simulink model "PiezoMPC2_17"  (R2022a)
settings: Solver=ode5  StartTime=0.0  StopTime=40  FixedStep=0.0001  RelTol=1e-3
values from neighbouring files (symbols this model uses):
  A = -1/tau    (= -1000)    [piezo_main.m]
  Abw = betas(7)    [StateFunction.m]    (also in piezo_main.m = 0.9)
  alpha = 80    [piezo_main.m]
  Aobs = [0, -B ... (first row only)    [piezo_main.m]
  B = 1/tau    (= 1000)    [piezo_main.m]
  beta1 = betas(1)    [StateFunction.m]    (also in piezo_main.m = 0.0032)
  beta2 = betas(2)    [StateFunction.m]    (also in piezo_main.m = 0.0035)
  beta3 = betas(3)    [StateFunction.m]    (also in piezo_main.m = -0.001)
  beta4 = betas(4)    [StateFunction.m]    (also in piezo_main.m = -0.0003)
  beta5 = betas(5)    [StateFunction.m]    (also in piezo_main.m = -0.0002)
  beta6 = betas(6)    [StateFunction.m]    (also in piezo_main.m = 0.0004)
  betas = [beta1;beta2;beta3;beta4;beta5;beta6;Abw;A;B;dp]    [piezo_main.m]
  C = [1, 0]    [piezo_main.m]
  dp = 1.6    [piezo_main.m]
  K = [10.0, 0.0 ... (first row only)    [piezo_main.m]
  kappa = 500    [piezo_main.m]
  S_inv = [  2*theta ,        -(1/B)*theta^2 ... (first row only)    [piezo_main.m]
undefined symbols (not defined in the file or in its folder): freq
libraries: mpclib x1
settings Model: Creator=CIO  LastModifiedBy=CIO
settings SolverCC: AlgebraicLoopSolver=TrustRegion
settings OptimizationCC: ZeroExternalMemoryAtStartup=off  ZeroInternalMemoryAtStartup=off  InitFltsAndDblsToZero=on
settings DebuggingCC: UnconnectedInputMsg=warning  UnconnectedOutputMsg=warning  UnconnectedLineMsg=warning  SFMachineParentedDataDiag=warning  ArithmeticOperatorsInVariantConditions=warning
settings HardwareCC: ProdLongLongMode=on  TargetLongLongMode=on
settings SFSimCC: CustomCodeUndefinedFunction=UseInterfaceOnly  SimTargetLang=C++
settings RTWCC: TargetLang=C++  DLArmComputeVersion=19.05
settings GRTTargetCC: TargetLangStandard=C++03 (ISO)  CodeInterfacePackaging=C++ class

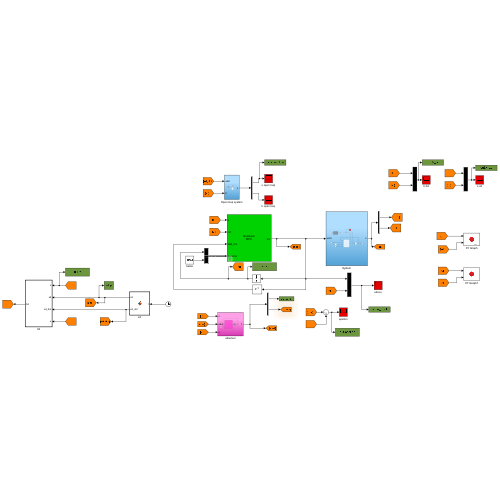
[thumbnail: Simulink's stored preview of the top-level diagram]
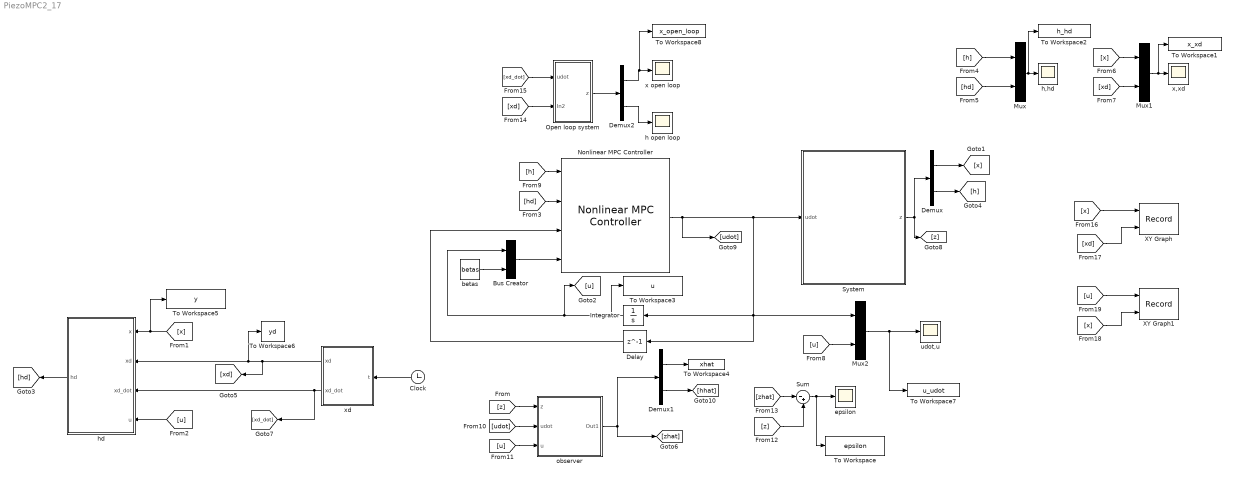
== system PiezoMPC2_17 ==
  Bus Creator : BusCreator  Inputs=2  OutDataTypeStr=Bus: myBusObject  NonVirtualBus=on
      settings: InheritFromInputs=off
  Clock : Clock
  Delay : Delay  DelayLength=1  InitialCondition=0
  Demux : Demux  Outputs=2
  Demux1 : Demux  Outputs=2
  Demux2 : Demux  Outputs=2
  Integrator : Integrator
  Mux : Mux  Inputs=2
  Mux1 : Mux  Inputs=2
  Mux2 : Mux  Inputs=2
  Nonlinear MPC Controller : mpclib/Nonlinear MPC Controller  SCDEnableBlockLinearizationSpecification=on  nlmpcobj=nlobj  UseObjectTs=on  UseMEX=off  md_enabled=off  mvtarget_enabled=off  param_enabled=on  cost_enabled=off  mvseq_enabled=off  stateseq_enabled=off  ovseq_enabled=off  slack_enabled=off  status_enabled=off  ov_min=off  ov_max=off  mv_min=off  mv_max=off  mvrate_min=off  mvrate_max=off  state_min=off  state_max=off  ov_weight=off  mv_weight=off  mvrate_weight=off  ecr_weight=off  nlp_initialize=off
  "Open loop system " : Subsystem
  Sum : Sum  Inputs=|-+
  System : Subsystem
  To Workspace : ToWorkspace  VariableName=epsilon  SampleTime=-1
  To Workspace1 : ToWorkspace  VariableName=x_xd  SampleTime=-1
  To Workspace2 : ToWorkspace  VariableName=h_hd  SampleTime=-1
  To Workspace3 : ToWorkspace  VariableName=u  SampleTime=-1
  To Workspace4 : ToWorkspace  VariableName=xhat  SampleTime=-1
  To Workspace5 : ToWorkspace  VariableName=y  SampleTime=-1
  To Workspace6 : ToWorkspace  VariableName=yd  SampleTime=-1
  To Workspace7 : ToWorkspace  VariableName=u_udot  SampleTime=-1
  To Workspace8 : ToWorkspace  VariableName=x_open_loop  SampleTime=-1
  XY Graph : Record  FileSettingsInternal="{\"entries\":[{\"content\":{\"excelSettings\":{\"content\":{},\"type\":\"Streamout.ExcelSettings\"}},\"type\":\"Streamout.FileSettingStorage\",\"uuid\":\"43ed1803-2e51-4bcb-b320-9c9d12944944\"}],\"packageUris\":[\"http://schema.mathworks.com/mf0/streamout_blocks/R2020a\"],\"version\":\"1.0\"}"  Layout=[1 1]  SignalsInternal="{\"entries\":[{\"content\":{\"signals\":[{\"content\":{\"blockPath\":[\"PiezoMPC2_17/XY Graph\"],\"channel\":[],\"dimensions\":[1],\"domain\":\"PiezoMPC2_17/XY Graph\",\"lineColor\":\"#a2142f\",\"plots\":[1],\"port\":1,\"sid\":[\"\"],\"signalID\":7776,\"signalName\":\"From16\"},\"type\":\"RecordBlkView.Signal\",\"uuid\":\"85c6ca8d-4860-42c1-af1f-82db8d25a64f\"},{\"content\":{\"blockPath\":[\"PiezoMPC2_17/XY Graph\"],\"channel\":[],\"dimensions\":[1],\"domain\":\"PiezoMPC2_17/XY Graph\",\"lineColor\":\"#139fff\",\"plots\":[1],\"port\":2,\"sid\":[\"\"],\"signalID\":7780,\"signalName\":\"From17\"},\"type\":\"RecordBlkView.Signal\",\"uuid\":\"68d22f8c-7fdf-4212-94fa-99e6d068a517\"}]},\"type\":\"RecordBlkView.InputSignals\",\"uuid\":\"7df4be47-02ba-4bd2-b1ad-eb6086c27650\"}],\"packageUris\":[\"http://schema.mathworks.com/mf0/streamout_blocks/R2020a\"],\"version\":\"1.0\"}"  VisualizationBindings="{\"xyplotplugin\":{\"info\":[{\"series\":[{\"bindingParametersList\":[{\"parameter\":\"X-Axis\",\"signalID\":7776,\"signalName\":\"From16\"},{\"parameter\":\"Y-Axis\",\"signalID\":7780,\"signalName\":\"From17\"}],\"seriesID\":32554}],\"subplotID\":1}]}}"  CompatibilityTag=XY
  XY Graph1 : Record  FileSettingsInternal="{\"entries\":[{\"content\":{\"excelSettings\":{\"content\":{},\"type\":\"Streamout.ExcelSettings\"}},\"type\":\"Streamout.FileSettingStorage\",\"uuid\":\"9b7f80d8-412e-4e2a-8833-cd9c8851424c\"}],\"packageUris\":[\"http://schema.mathworks.com/mf0/streamout_blocks/R2020a\"],\"version\":\"1.0\"}"  Layout=[1 1]  SignalsInternal="{\"entries\":[{\"content\":{\"signals\":[{\"content\":{\"blockPath\":[\"PiezoMPC2_17/XY Graph1\"],\"channel\":[],\"dimensions\":[1,1],\"domain\":\"PiezoMPC2_17/XY Graph1\",\"lineColor\":\"#a2142f\",\"plots\":[1],\"port\":1,\"sid\":[\"\"],\"signalID\":7784,\"signalName\":\"From19\"},\"type\":\"RecordBlkView.Signal\",\"uuid\":\"d37f6522-71ed-4229-9050-82b4d9bbd21d\"},{\"content\":{\"blockPath\":[\"PiezoMPC2_17/XY Graph1\"],\"channel\":[],\"dimensions\":[1],\"domain\":\"PiezoMPC2_17/XY Graph1\",\"lineColor\":\"#139fff\",\"plots\":[1],\"port\":2,\"sid\":[\"\"],\"signalID\":7788,\"signalName\":\"From18\"},\"type\":\"RecordBlkView.Signal\",\"uuid\":\"deba607d-0966-4bfa-aa24-ff5771058220\"}]},\"type\":\"RecordBlkView.InputSignals\",\"uuid\":\"5f0caead-39a7-4f6e-b661-079760aac763\"}],\"packageUris\":[\"http://schema.mathworks.com/mf0/streamout_blocks/R2020a\"],\"version\":\"1.0\"}"  VisualizationBindings="{\"xyplotplugin\":{\"info\":[{\"series\":[{\"bindingParametersList\":[{\"parameter\":\"X-Axis\",\"signalID\":7784,\"signalName\":\"From19\"},{\"parameter\":\"Y-Axis\",\"signalID\":7788,\"signalName\":\"From18\"}],\"seriesID\":21478}],\"subplotID\":1}]}}"  CompatibilityTag=XY
  betas : Constant  Value=betas  VectorParams1D=off
  epsilon : Scope
  h open loop : Scope
  h,hd : Scope
  hd : MATLAB Function  TreatAsAtomicUnit=on
  observer : Subsystem
  udot,u : Scope
  x open loop : Scope
  x,xd : Scope
  xd : MATLAB Function  TreatAsAtomicUnit=on
  wires:
  Bus Creator/1 -> Nonlinear MPC Controller/4
  betas/1 -> Bus Creator/2
  Nonlinear MPC Controller/1 -> Integrator/1, Mux2/1, Delay/1, System/1(udot), [udot]
  Delay/1 -> Nonlinear MPC Controller/3
  Integrator/1 -> To Workspace3/1, [u], Bus Creator/1
  System/1(z) -> Demux/1, [z]
  xd/2(xd_dot) -> [xd_dot], hd/3(xd_dot)
  xd/1(xd) -> [xd], To Workspace6/1, hd/2(xd)
  Clock/1 -> xd/1(t)
  [x] -> To Workspace5/1, hd/1(x)
  [u] -> hd/4(u)
  hd/1(hd) -> [hd]
  [h] -> Mux/1
  [hd] -> Mux/2
  Mux/1 -> To Workspace2/1, h,hd/1
  Mux1/1 -> To Workspace1/1, x,xd/1
  [x] -> Mux1/1
  [xd] -> Mux1/2
  Mux2/1 -> To Workspace7/1, udot,u/1
  [u] -> Mux2/2
  Demux/2 -> [h]
  Demux/1 -> [x]
  [h] -> Nonlinear MPC Controller/1
  [hd] -> Nonlinear MPC Controller/2
  [udot] -> observer/2(udot)
  [z] -> observer/1(z)
  observer/1(Out1) -> Demux1/1, [zhat]
  [u] -> observer/3(u)
  Demux1/1 -> To Workspace4/1
  Demux1/2 -> [hhat]
  [z] -> Sum/2
  Sum/1 -> To Workspace/1, epsilon/1
  [zhat] -> Sum/1
  "Open loop system "/1(z) -> Demux2/1
  [xd_dot] -> "Open loop system "/1(udot)
  [xd] -> "Open loop system "/2(In2)
  Demux2/2 -> h open loop/1
  Demux2/1 -> To Workspace8/1, x open loop/1
  [x] -> XY Graph/1
  [xd] -> XY Graph/2
  [x] -> XY Graph1/2
  [u] -> XY Graph1/1

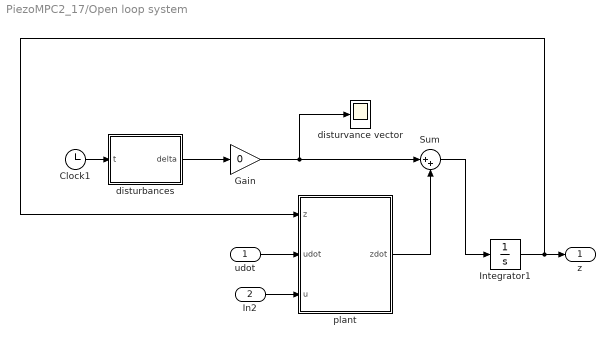
== system PiezoMPC2_17/Open loop system  ==
  udot : Inport
  In2 : Inport  Port=2
  Clock1 : Clock
  Gain : Gain  Gain=0
  Integrator1 : Integrator  InitialCondition="[3  -2]"
  Sum : Sum  Inputs=|++
  disturbances : MATLAB Function  TreatAsAtomicUnit=on
  disturvance vector : Scope
  plant : MATLAB Function  TreatAsAtomicUnit=on
  z : Outport
  wires:
  Integrator1/1 -> z/1, plant/1(z)
  udot/1 -> plant/2(udot)
  In2/1 -> plant/3(u)
  Gain/1 -> Sum/1, disturvance vector/1
  disturbances/1(delta) -> Gain/1
  plant/1(zdot) -> Sum/2
  Clock1/1 -> disturbances/1(t)
  Sum/1 -> Integrator1/1

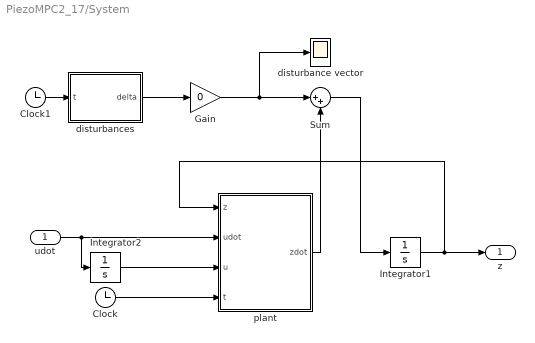
== system PiezoMPC2_17/System ==
  udot : Inport
  Clock : Clock
  Clock1 : Clock
  Gain : Gain  Gain=0
  Integrator1 : Integrator  InitialCondition="[3  -2]"
  Integrator2 : Integrator
  Sum : Sum  Inputs=|++
  disturbance vector : Scope
  disturbances : MATLAB Function  TreatAsAtomicUnit=on
  plant : MATLAB Function  TreatAsAtomicUnit=on
  z : Outport
  wires:
  udot/1 -> Integrator2/1, plant/2(udot)
  Integrator1/1 -> z/1, plant/1(z)
  Integrator2/1 -> plant/3(u)
  Clock/1 -> plant/4(t)
  Gain/1 -> Sum/1, disturbance vector/1
  disturbances/1(delta) -> Gain/1
  Sum/1 -> Integrator1/1
  plant/1(zdot) -> Sum/2
  Clock1/1 -> disturbances/1(t)

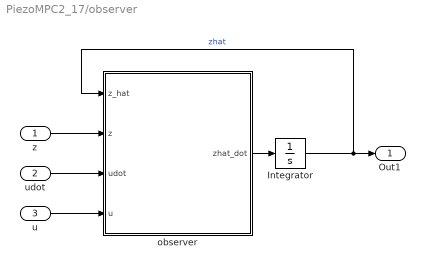
== system PiezoMPC2_17/observer ==
  z : Inport
  udot : Inport  Port=2
  u : Inport  Port=3
  Integrator : Integrator  InitialCondition=[0;0]
  observer : MATLAB Function  TreatAsAtomicUnit=on
  Out1 : Outport  VectorParamsAs1DForOutWhenUnconnected=off
  wires:
  observer/1(zhat_dot) -> Integrator/1
  Integrator/1 -> observer/1(z_hat), Out1/1  "zhat"
  z/1 -> observer/2(z)
  udot/1 -> observer/3(udot)
  u/1 -> observer/4(u)

== matlab function PiezoMPC2_17/Open loop system /disturbances ==
  data: t input; delta output
function delta = dist(t)

delta_x = 30;
delta_h = 25*sin(t); %2*sin(t); -- causa error en el observer

delta = [delta_x ; delta_h];

== matlab function PiezoMPC2_17/System/disturbances ==
  data: t input; delta output
function delta = dist(t)

delta_x = 30;
delta_h = 25*sin(t); 

delta = [delta_x ; delta_h];

== matlab function PiezoMPC2_17/observer/observer ==
  data: z_hat input; z input; udot input; u input; Aobs parameter; Abw parameter; zhat_dot output; A parameter; B parameter; dp parameter; S_inv parameter; C parameter; beta1 parameter; beta2 parameter; beta3 parameter; beta4 parameter; beta5 parameter; beta6 parameter; K parameter
function zhat_dot = obs(z_hat, z, udot, u, Aobs, Abw, A, B, dp,S_inv, C, ...
                        beta1, beta2, beta3, beta4, beta5, beta6,K)
    

    h_hat     = z_hat(2);
    x_hat     = z_hat(1);           
    
    Phi = beta1*sign( udot*h_hat ) + beta2*sign( udot*u ) + ...
          beta3*sign( u*h_hat )    + beta4*sign( udot )   + ...
          beta5*sign( h_hat )      + beta6*sign( u );
      
    gx = [ A*x_hat + B*dp*u ; 
           udot*( Abw - abs(h_hat)*Phi )];


    epsilon = z_hat - z;
    zhat_dot = Aobs*z_hat + gx - S_inv*(C)'*C*epsilon -  S_inv*K*(C)'*C*sign(epsilon) ;

end

== matlab function PiezoMPC2_17/System/plant ==
  data: z input; udot input; u input; zdot output; beta1 parameter; beta2 parameter; beta3 parameter; beta4 parameter; beta5 parameter; beta6 parameter; Abw parameter; A parameter; B parameter; dp parameter; t input
function zdot = fcn(z,udot,u,beta1, beta2, beta3, beta4, beta5, beta6, Abw, A, B, dp,t)

    %States
    h     = z(2);
    x     = z(1);           
    
    Phi = beta1*sign( udot*h ) + beta2*sign( udot*u ) + ...
          beta3*sign( u*h )    + beta4*sign( udot )   + ...
          beta5*sign( h )      + beta6*sign( u );
      
    zdot = zeros(2,1);
    %============================ System model ============================
    %xdot
    zdot(1) = A*x + B*(dp*u - h);
    
    %hdot
    zdot(2) = udot*( Abw - abs(h)*Phi );
    
end

== matlab function PiezoMPC2_17/hd ==
  data: x input; xd input; xd_dot input; u input; hd output; A parameter; B parameter; kappa parameter; dp parameter
function hd = fcn(x,xd,xd_dot,u, A, B, kappa, dp)

    xtes = x - xd;
    hd   = (1/B)*( (A - kappa)*xtes + A*xd - xd_dot + B*dp*u );

end

== matlab function PiezoMPC2_17/xd ==
  data: t input; xd output; xd_dot output; alpha parameter; freq parameter
function [xd, xd_dot] = fcn(t,alpha, freq)

	xd     = alpha*sin(freq*t);
    xd_dot = alpha*cos(freq*t);
end

== matlab function PiezoMPC2_17/Open loop system /plant ==
  data: z input; udot input; u input; zdot output; beta1 parameter; beta2 parameter; beta3 parameter; beta4 parameter; beta5 parameter; beta6 parameter; Abw parameter; A parameter; B parameter; dp parameter
function zdot = fcn(z,udot,u,beta1, beta2, beta3, beta4, beta5, beta6, Abw, A, B, dp)

    %States
    h     = z(2);
    x     = z(1);           
    
    Phi = beta1*sign( udot*h ) + beta2*sign( udot*u ) + ...
          beta3*sign( u*h )    + beta4*sign( udot )   + ...
          beta5*sign( h )      + beta6*sign( u );
      
    zdot = zeros(2,1);
    %============================ System model ============================
    %xdot
    zdot(1) = A*x + B*(dp*u - h);
    
    %hdot
    zdot(2) = udot*( Abw - abs(h)*Phi );
    
end
